simulink model "exampleAbsoChiller"  (Simulink 7.6)
settings: Solver=ode45  StartTime=0.0  StopTime=10*3600  RelTol=1e-3
libraries: carnot x4
settings Model: Creator=drhf  LastModifiedBy=drhf
settings CodeAppCC: CustomSymbolStrType=$N$R$M_T

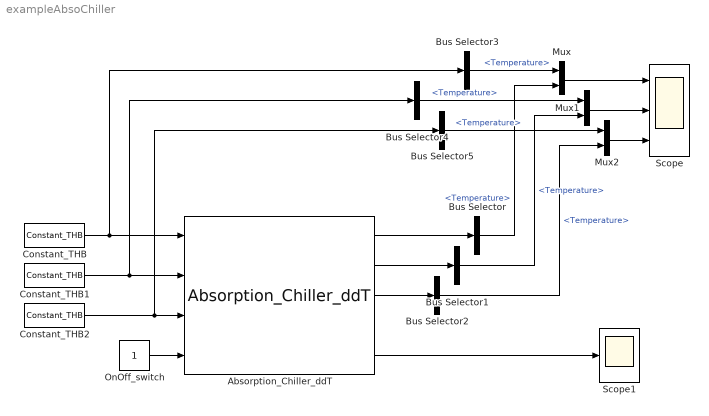
== system exampleAbsoChiller ==
  Absorption_Chiller_ddT : carnot/Source/Chiller/Absorption_Chiller_ddT  SystemSampleTime=-1  E=1.2  sE=0.42  rE=0.9  sG=0.51  rG=2/0.51  dpe=[100 1e4]  dpg=[100 1e4]  Pel_p=80
  Bus Selector{,1..5} (6 alike) : BusSelector  OutputSignals=Temperature
  Constant_THB : carnot/Source/Simple/Constant_THB  SystemSampleTime=-1  t=15  mdot=1200/3600  p=1e5  mID=No Pressure Drop  fluid=water  mix=0  dia=0.02  hgt=0
  Constant_THB1 : carnot/Source/Simple/Constant_THB  SystemSampleTime=-1  t=90  mdot=1200/3600  p=1e5  mID=No Pressure Drop  fluid=water  mix=0  dia=0.02  hgt=0
  Constant_THB2 : carnot/Source/Simple/Constant_THB  SystemSampleTime=-1  t=30  mdot=1200/3600  p=1e5  mID=No Pressure Drop  fluid=water  mix=0  dia=0.02  hgt=0
  Mux : Mux  Inputs=2
  Mux1 : Mux  Inputs=2
  Mux2 : Mux  Inputs=2
  OnOff_switch : Constant
      settings: OpenFcn=set_param(gcb,'value',num2str(1-str2num(get_param(gcb,'value'))))
  Scope : Scope  NumInputPorts=3
      settings: YMin=-5~-5~-5  YMax=5~5~5
  Scope1 : Scope
  wires:
  Constant_THB/1 -> Bus Selector3/1, Absorption_Chiller_ddT/1
  Constant_THB1/1 -> Bus Selector4/1, Absorption_Chiller_ddT/2
  Constant_THB2/1 -> Bus Selector5/1, Absorption_Chiller_ddT/3
  OnOff_switch/1 -> Absorption_Chiller_ddT/4
  Absorption_Chiller_ddT/1 -> Bus Selector/1
  Bus Selector/1 -> Mux/2  "<Temperature>"
  Absorption_Chiller_ddT/2 -> Bus Selector1/1
  Bus Selector1/1 -> Mux1/2  "<Temperature>"
  Absorption_Chiller_ddT/3 -> Bus Selector2/1
  Bus Selector2/1 -> Mux2/2  "<Temperature>"
  Bus Selector3/1 -> Mux/1  "<Temperature>"
  Mux/1 -> Scope/1
  Mux1/1 -> Scope/2
  Bus Selector4/1 -> Mux1/1  "<Temperature>"
  Mux2/1 -> Scope/3
  Bus Selector5/1 -> Mux2/1  "<Temperature>"
  Absorption_Chiller_ddT/5 -> Scope1/1
